simulink model "UC613_1"  (R2022b)
settings: Solver=VariableStepAuto  StartTime=0.0  StopTime=10.0  RelTol=1e-3
model workspace (MAT data in the model file):
  DataStorageSize = Simulink.Parameter
  DataStorageSize.DataType = 'uint16'
  DataStorageSize.DocUnits = 'GB'
  DataStorageSize.Complexity = 'real'
  DataStorageSize.Dimensions = [0 0]
settings Model: ParameterArgumentNames=DataStorageSize  Creator=TO41629  LastModifiedBy=TO41629

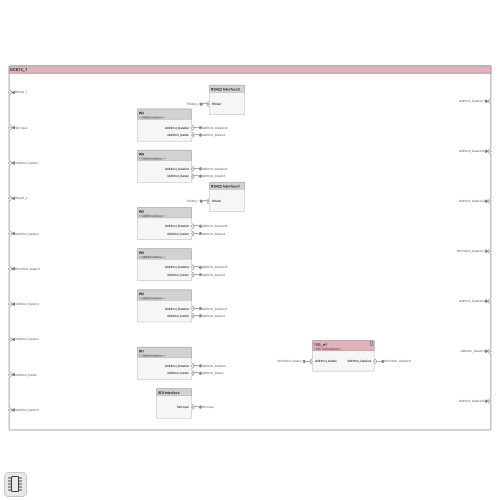
[thumbnail: Simulink's stored preview of the top-level diagram]
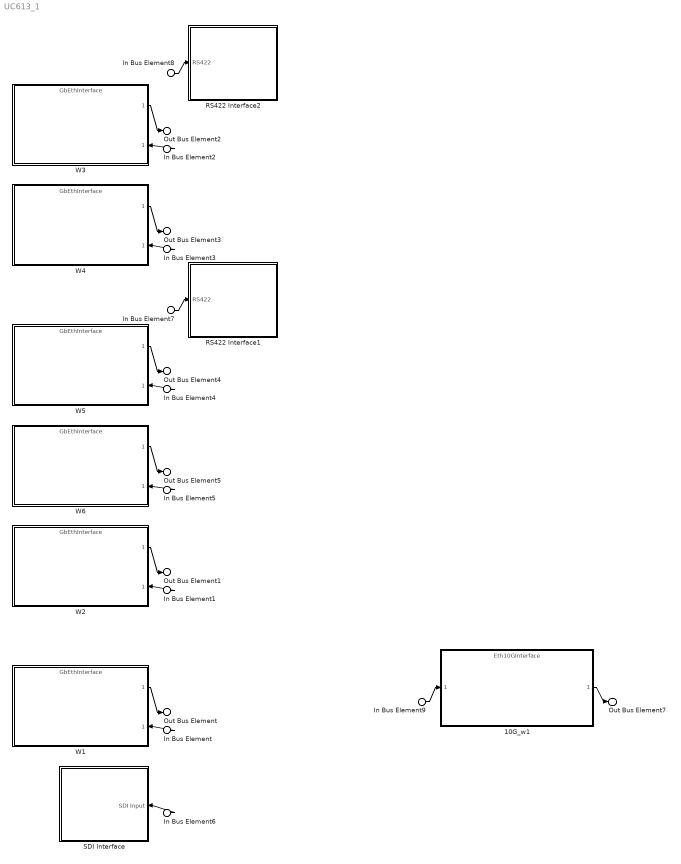
== system UC613_1 ==
  In Bus Element7 : Inport  PortName=RS422_1
  In Bus Element6 : Inport  Port=2  PortName=SDI Input
  In Bus Element1 : Inport  Port=3  PortName=GbEthInt_DataIn1
  In Bus Element8 : Inport  Port=4  PortName=RS422_2
  In Bus Element2 : Inport  Port=5  PortName=GbEthInt_DataIn2
  In Bus Element9 : Inport  Port=6  PortName=Eth10GInt_DataIn1
  In Bus Element3 : Inport  Port=7  PortName=GbEthInt_DataIn3
  In Bus Element4 : Inport  Port=8  PortName=GbEthInt_DataIn4
  In Bus Element : Inport  Port=9  PortName=GbEthInt_DataIn
  In Bus Element5 : Inport  Port=10  PortName=GbEthInt_DataIn5
  10G_w1 : ModelReference  ModelNameDialog=Eth10GInterface  UsingDefaultArgumentValue=0,0,0  SimulationMode=Normal  ModelReferenceVersion=1.28
      settings: PortSchema="{\"entries\":[{\"content\":{\"headerSize\":38,\"margin\":15,\"minimumSpacing\":25,\"sides\":[{\"content\":{\"connectorIds\":[\"In1\"]},\"type\":\"ConnectorPlacement.EquallySpacedRectSide\",\"uuid\":\"c7a9dcc5-4699-4aa5-9b03-01cd9c9d5d35\"},{\"content\":{\"connectorIds\":[\"Out1\"],\"side\":\"RIGHT\"},\"type\":\"ConnectorPlacement.EquallySpacedRectSide\",\"uuid\":\"7085d3c2-4a9c-4f60-a450-73088e37e883\"},{\"content\":{\"connectorIds\":[],\"side\":\"TOP\"},\"type\":\"ConnectorPlacement.EquallySpacedRectSide\",\"uuid\":\"b1aea649-404c-4f50-816f-0908c9ccfd50\"}]},\"type\":\"ConnectorPlacement.EquallySpacedConnector\",\"uuid\":\"4d292e22-38cf-4a1e-b63b-51fd039b5bd2\"}],\"packageUris\":[\"http://schema.mathworks.com/mf0/Connector/R2020b\"],\"version\":\"1.0\"}"
  RS422 Interface1 : Subsystem
      settings: PortSchema="{\"entries\":[{\"content\":{\"headerSize\":26,\"margin\":15,\"minimumSpacing\":25,\"sides\":[{\"content\":{\"connectorIds\":[\"In1\"]},\"type\":\"ConnectorPlacement.EquallySpacedRectSide\",\"uuid\":\"c7a9dcc5-4699-4aa5-9b03-01cd9c9d5d35\"},{\"content\":{\"connectorIds\":[],\"side\":\"RIGHT\"},\"type\":\"ConnectorPlacement.EquallySpacedRectSide\",\"uuid\":\"7085d3c2-4a9c-4f60-a450-73088e37e883\"},{\"content\":{\"connectorIds\":[],\"side\":\"TOP\"},\"type\":\"ConnectorPlacement.EquallySpacedRectSide\",\"uuid\":\"b1aea649-404c-4f50-816f-0908c9ccfd50\"}]},\"type\":\"ConnectorPlacement.EquallySpacedConnector\",\"uuid\":\"4d292e22-38cf-4a1e-b63b-51fd039b5bd2\"}],\"packageUris\":[\"http://schema.mathworks.com/mf0/Connector/R2020b\"],\"version\":\"1.0\"}"
  RS422 Interface2 : Subsystem
      settings: PortSchema="{\"entries\":[{\"content\":{\"headerSize\":26,\"margin\":15,\"minimumSpacing\":25,\"sides\":[{\"content\":{\"connectorIds\":[\"In1\"]},\"type\":\"ConnectorPlacement.EquallySpacedRectSide\",\"uuid\":\"c7a9dcc5-4699-4aa5-9b03-01cd9c9d5d35\"},{\"content\":{\"connectorIds\":[],\"side\":\"RIGHT\"},\"type\":\"ConnectorPlacement.EquallySpacedRectSide\",\"uuid\":\"7085d3c2-4a9c-4f60-a450-73088e37e883\"},{\"content\":{\"connectorIds\":[],\"side\":\"TOP\"},\"type\":\"ConnectorPlacement.EquallySpacedRectSide\",\"uuid\":\"b1aea649-404c-4f50-816f-0908c9ccfd50\"}]},\"type\":\"ConnectorPlacement.EquallySpacedConnector\",\"uuid\":\"4d292e22-38cf-4a1e-b63b-51fd039b5bd2\"}],\"packageUris\":[\"http://schema.mathworks.com/mf0/Connector/R2020b\"],\"version\":\"1.0\"}"
  SDI Interface : Subsystem
      settings: PortSchema="{\"entries\":[{\"content\":{\"headerSize\":26,\"margin\":15,\"minimumSpacing\":25,\"sides\":[{\"content\":{\"connectorIds\":[]},\"type\":\"ConnectorPlacement.EquallySpacedRectSide\",\"uuid\":\"c7a9dcc5-4699-4aa5-9b03-01cd9c9d5d35\"},{\"content\":{\"connectorIds\":[\"In1\"],\"side\":\"RIGHT\"},\"type\":\"ConnectorPlacement.EquallySpacedRectSide\",\"uuid\":\"7085d3c2-4a9c-4f60-a450-73088e37e883\"},{\"content\":{\"connectorIds\":[],\"side\":\"TOP\"},\"type\":\"ConnectorPlacement.EquallySpacedRectSide\",\"uuid\":\"b1aea649-404c-4f50-816f-0908c9ccfd50\"}]},\"type\":\"ConnectorPlacement.EquallySpacedConnector\",\"uuid\":\"4d292e22-38cf-4a1e-b63b-51fd039b5bd2\"}],\"packageUris\":[\"http://schema.mathworks.com/mf0/Connector/R2020b\"],\"version\":\"1.0\"}"
  W{1..6} (6 alike) : ModelReference  ModelNameDialog=GbEthInterface  UsingDefaultArgumentValue=0,0,0  SimulationMode=Normal  ModelReferenceVersion=1.28
      settings: PortSchema="{\"entries\":[{\"content\":{\"headerSize\":38,\"margin\":15,\"minimumSpacing\":25,\"sides\":[{\"content\":{\"connectorIds\":[]},\"type\":\"ConnectorPlacement.EquallySpacedRectSide\",\"uuid\":\"c7a9dcc5-4699-4aa5-9b03-01cd9c9d5d35\"},{\"content\":{\"connectorIds\":[\"Out1\",\"In1\"],\"side\":\"RIGHT\"},\"type\":\"ConnectorPlacement.EquallySpacedRectSide\",\"uuid\":\"7085d3c2-4a9c-4f60-a450-73088e37e883\"},{\"content\":{\"connectorIds\":[],\"side\":\"TOP\"},\"type\":\"ConnectorPlacement.EquallySpacedRectSide\",\"uuid\":\"b1aea649-404c-4f50-816f-0908c9ccfd50\"}]},\"type\":\"ConnectorPlacement.EquallySpacedConnector\",\"uuid\":\"4d292e22-38cf-4a1e-b63b-51fd039b5bd2\"}],\"packageUris\":[\"http://schema.mathworks.com/mf0/Connector/R2020b\"],\"version\":\"1.0\"}"
  Out Bus Element1 : Outport  PortName=GbEthInt_DataOut1
  Out Bus Element2 : Outport  Port=2  PortName=GbEthInt_DataOut2
  Out Bus Element3 : Outport  Port=3  PortName=GbEthInt_DataOut3
  Out Bus Element7 : Outport  Port=4  PortName=Eth10GInt_DataOut1
  Out Bus Element4 : Outport  Port=5  PortName=GbEthInt_DataOut4
  Out Bus Element : Outport  Port=6  PortName=GbEthInt_DataOut
  Out Bus Element5 : Outport  Port=7  PortName=GbEthInt_DataOut5
  wires:
  In Bus Element7/1 -> RS422 Interface1/1(RS422)
  In Bus Element8/1 -> RS422 Interface2/1(RS422)
  W6/1 -> Out Bus Element5/1
  W5/1 -> Out Bus Element4/1
  W4/1 -> Out Bus Element3/1
  W3/1 -> Out Bus Element2/1
  In Bus Element9/1 -> 10G_w1/1
  W2/1 -> Out Bus Element1/1
  W1/1 -> Out Bus Element/1
  In Bus Element/1 -> W1/1
  In Bus Element1/1 -> W2/1
  In Bus Element2/1 -> W3/1
  In Bus Element5/1 -> W6/1
  In Bus Element4/1 -> W5/1
  In Bus Element3/1 -> W4/1
  In Bus Element6/1 -> SDI Interface/1(SDI Input)
  10G_w1/1 -> Out Bus Element7/1

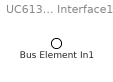
== system UC613_1/RS422 Interface1 ==
  Bus Element In1 : Inport  PortName=RS422

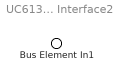
== system UC613_1/RS422 Interface2 ==
  Bus Element In1 : Inport  PortName=RS422

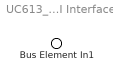
== system UC613_1/SDI Interface ==
  Bus Element In1 : Inport  PortName=SDI Input
